simulink model "Task_8_Rlung"  (R2015a)
settings: Solver=ode45  StartTime=0.0  StopTime=10.0  RelTol=1e-3
libraries: simulink x2
settings Model: Creator=Farhan Fuad  LastModifiedBy=Farhan Fuad

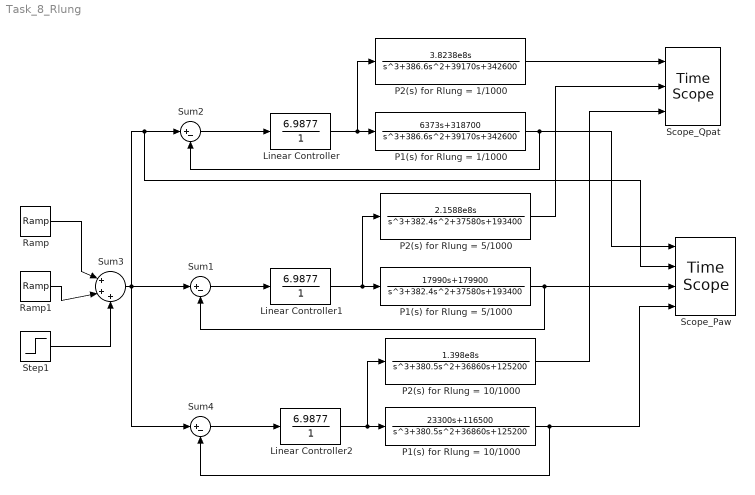
== system Task_8_Rlung ==
  Linear Controller : TransferFcn  Numerator=[6.9877]  Denominator=[1 ]
  Linear Controller1 : TransferFcn  Numerator=[6.9877]  Denominator=[1 ]
  Linear Controller2 : TransferFcn  Numerator=[6.9877]  Denominator=[1 ]
  P1(s) for Rlung = 1/1000 : TransferFcn  Numerator=[0 0 6373 318700]  Denominator=[1 386.6 39170 342600]
  P1(s) for Rlung = 10/1000 : TransferFcn  Numerator=[0 0 23300 116500]  Denominator=[1 380.5 36860 125200]
  P1(s) for Rlung = 5/1000 : TransferFcn  Numerator=[0 0 17990 179900]  Denominator=[1 382.4 37580 193400]
  P2(s) for Rlung = 1/1000 : TransferFcn  Numerator=[0 0 3.8238e8 0]  Denominator=[1 386.6 39170 342600]
  P2(s) for Rlung = 10/1000 : TransferFcn  Numerator=[0 0 1.398e8 0]  Denominator=[1 380.5 36860 125200]
  P2(s) for Rlung = 5/1000 : TransferFcn  Numerator=[0 0 2.1588e8 0]  Denominator=[1 382.4 37580 193400]
  Ramp : simulink/Sources/Ramp  slope=64.865  start=1  X0=0
  Ramp1 : simulink/Sources/Ramp  slope=-64.865  start=1.23125  X0=0
  "Scope_Paw " : TimeScope  NumInputPorts=4
  Scope_Qpat : TimeScope  NumInputPorts=3
  Step1 : Step  Time=5  After=-15  SampleTime=0
  Sum1 : Sum  Inputs=|+-
  Sum2 : Sum  Inputs=|+-
  Sum3 : Sum  Inputs=|+++
  Sum4 : Sum  Inputs=|+-
  wires:
  Ramp/1 -> Sum3/1
  Ramp1/1 -> Sum3/2
  Sum2/1 -> Linear Controller/1
  P2(s) for Rlung = 1/1000/1 -> Scope_Qpat/1
  P1(s) for Rlung = 1/1000/1 -> "Scope_Paw "/1, Sum2/2
  Step1/1 -> Sum3/3
  Linear Controller/1 -> P2(s) for Rlung = 1/1000/1, P1(s) for Rlung = 1/1000/1
  Sum1/1 -> Linear Controller1/1
  P2(s) for Rlung = 5/1000/1 -> Scope_Qpat/2
  P1(s) for Rlung = 5/1000/1 -> Sum1/2, "Scope_Paw "/3
  Linear Controller1/1 -> P1(s) for Rlung = 5/1000/1, P2(s) for Rlung = 5/1000/1
  Sum4/1 -> Linear Controller2/1
  Sum3/1 -> "Scope_Paw "/2, Sum2/1, Sum4/1, Sum1/1
  P1(s) for Rlung = 10/1000/1 -> Sum4/2, "Scope_Paw "/4
  Linear Controller2/1 -> P2(s) for Rlung = 10/1000/1, P1(s) for Rlung = 10/1000/1
  P2(s) for Rlung = 10/1000/1 -> Scope_Qpat/3
